simulink model "TST_PthSet_TrqCalc"  (R2016b)
settings: Solver=FixedStepDiscrete  StartTime=0.0  StopTime=simTime  FixedStep=sampleTime  RelTol=1e-3
values from neighbouring files (symbols this model uses):
  testCase = 1    [initTST_PthSet_TrqCalc_001.m]    (also in initTST_PthSet_TrqCalc_002.m = 2; initTST_PthSet_TrqCalc_003.m = 3)
libraries: simulink x17, UnitTest_Lib x12
settings Model: Creator=zhengjinyan  LastModifiedBy=zhengjinyan
settings DebuggingCC: SignalRangeChecking=error

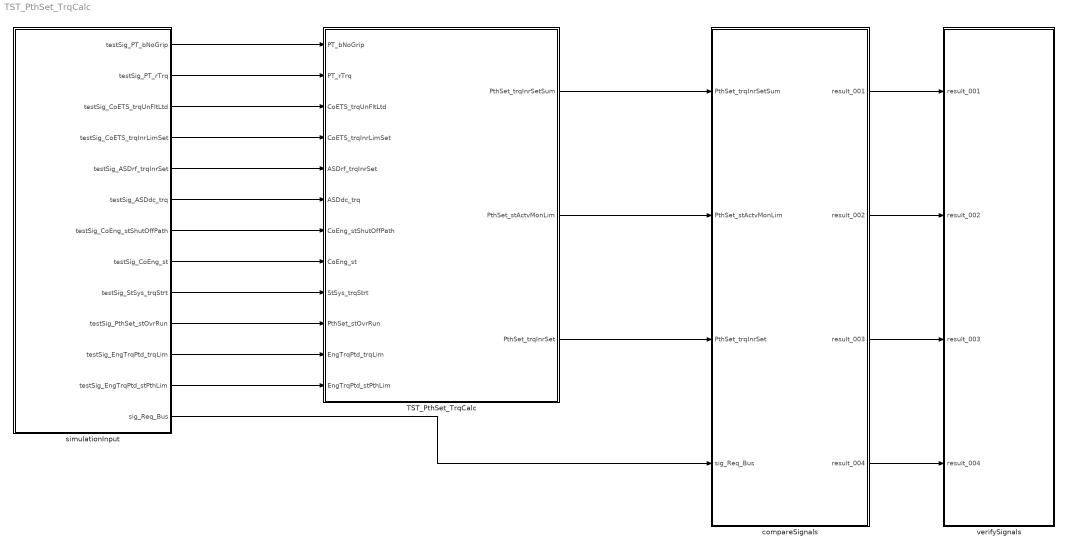
== system TST_PthSet_TrqCalc ==
  TST_PthSet_TrqCalc : Subsystem
  compareSignals : Subsystem
  simulationInput : Subsystem
  verifySignals : Subsystem
  wires:
  simulationInput/1(testSig_PT_bNoGrip) -> TST_PthSet_TrqCalc/1(PT_bNoGrip)
  simulationInput/2(testSig_PT_rTrq) -> TST_PthSet_TrqCalc/2(PT_rTrq)
  simulationInput/3(testSig_CoETS_trqUnFltLtd) -> TST_PthSet_TrqCalc/3(CoETS_trqUnFltLtd)
  simulationInput/4(testSig_CoETS_trqInrLimSet) -> TST_PthSet_TrqCalc/4(CoETS_trqInrLimSet)
  simulationInput/5(testSig_ASDrf_trqInrSet) -> TST_PthSet_TrqCalc/5(ASDrf_trqInrSet)
  simulationInput/6(testSig_ASDdc_trq) -> TST_PthSet_TrqCalc/6(ASDdc_trq)
  simulationInput/7(testSig_CoEng_stShutOffPath) -> TST_PthSet_TrqCalc/7(CoEng_stShutOffPath)
  simulationInput/8(testSig_CoEng_st) -> TST_PthSet_TrqCalc/8(CoEng_st)
  simulationInput/9(testSig_StSys_trqStrt) -> TST_PthSet_TrqCalc/9(StSys_trqStrt)
  simulationInput/10(testSig_PthSet_stOvrRun) -> TST_PthSet_TrqCalc/10(PthSet_stOvrRun)
  simulationInput/11(testSig_EngTrqPtd_trqLim) -> TST_PthSet_TrqCalc/11(EngTrqPtd_trqLim)
  simulationInput/12(testSig_EngTrqPtd_stPthLim) -> TST_PthSet_TrqCalc/12(EngTrqPtd_stPthLim)
  TST_PthSet_TrqCalc/1(PthSet_trqInrSetSum) -> compareSignals/1(PthSet_trqInrSetSum)
  TST_PthSet_TrqCalc/2(PthSet_stActvMonLim) -> compareSignals/2(PthSet_stActvMonLim)
  TST_PthSet_TrqCalc/3(PthSet_trqInrSet) -> compareSignals/3(PthSet_trqInrSet)
  simulationInput/13(sig_Req_Bus) -> compareSignals/4(sig_Req_Bus)
  compareSignals/1(result_001) -> verifySignals/1(result_001)
  compareSignals/2(result_002) -> verifySignals/2(result_002)
  compareSignals/3(result_003) -> verifySignals/3(result_003)
  compareSignals/4(result_004) -> verifySignals/4(result_004)

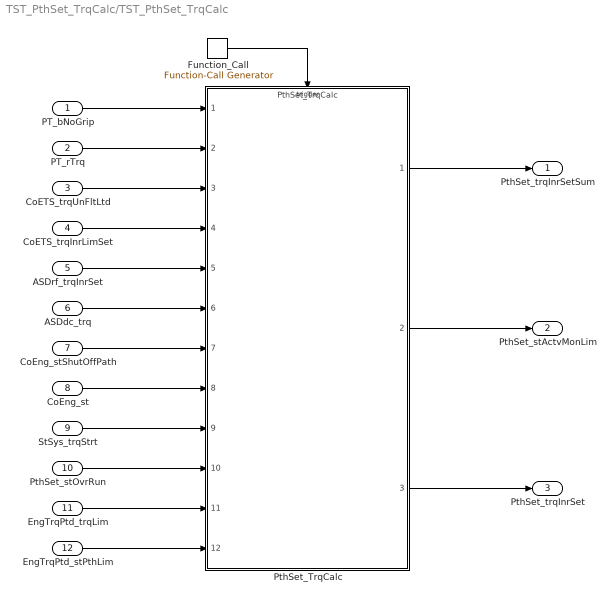
== system TST_PthSet_TrqCalc/TST_PthSet_TrqCalc ==
  PT_bNoGrip : Inport
  PT_rTrq : Inport  Port=2
  CoETS_trqUnFltLtd : Inport  Port=3
  CoETS_trqInrLimSet : Inport  Port=4
  ASDrf_trqInrSet : Inport  Port=5
  ASDdc_trq : Inport  Port=6
  CoEng_stShutOffPath : Inport  Port=7
  CoEng_st : Inport  Port=8
  StSys_trqStrt : Inport  Port=9
  PthSet_stOvrRun : Inport  Port=10
  EngTrqPtd_trqLim : Inport  Port=11
  EngTrqPtd_stPthLim : Inport  Port=12
  Function_Call : simulink/Ports & Subsystems/Function-Call Generator  sample_time=sampleTime  numberOfIterations=1
  PthSet_TrqCalc : ModelReference  ModelNameDialog=PthSet_TrqCalc  SimulationMode=Normal  ModelReferenceVersion=1.11  TriggerPortName=function  TriggerPortTriggerType=function-call  TriggerPortStatesWhenEnabling=held
  PthSet_trqInrSetSum : Outport
  PthSet_stActvMonLim : Outport  Port=2
  PthSet_trqInrSet : Outport  Port=3
  wires:
  Function_Call/1 -> PthSet_TrqCalc/Trigger
  PT_bNoGrip/1 -> PthSet_TrqCalc/1
  PT_rTrq/1 -> PthSet_TrqCalc/2
  CoETS_trqUnFltLtd/1 -> PthSet_TrqCalc/3
  CoETS_trqInrLimSet/1 -> PthSet_TrqCalc/4
  ASDrf_trqInrSet/1 -> PthSet_TrqCalc/5
  ASDdc_trq/1 -> PthSet_TrqCalc/6
  CoEng_stShutOffPath/1 -> PthSet_TrqCalc/7
  CoEng_st/1 -> PthSet_TrqCalc/8
  StSys_trqStrt/1 -> PthSet_TrqCalc/9
  PthSet_stOvrRun/1 -> PthSet_TrqCalc/10
  EngTrqPtd_trqLim/1 -> PthSet_TrqCalc/11
  EngTrqPtd_stPthLim/1 -> PthSet_TrqCalc/12
  PthSet_TrqCalc/1 -> PthSet_trqInrSetSum/1
  PthSet_TrqCalc/2 -> PthSet_stActvMonLim/1
  PthSet_TrqCalc/3 -> PthSet_trqInrSet/1

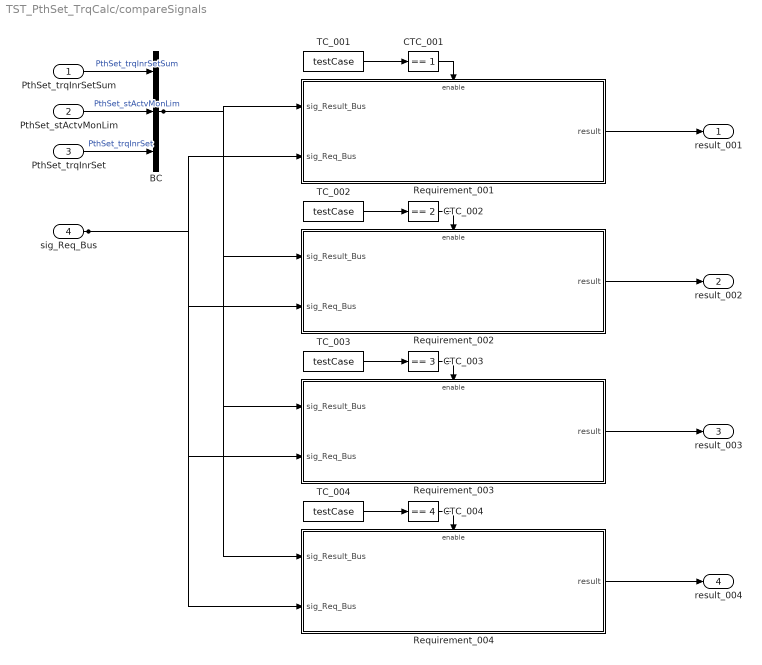
== system TST_PthSet_TrqCalc/compareSignals ==
  PthSet_trqInrSetSum : Inport
  PthSet_stActvMonLim : Inport  Port=2
  PthSet_trqInrSet : Inport  Port=3
  sig_Req_Bus : Inport  Port=4
  BC : BusCreator  Inputs=3
  CTC_001 : simulink/Logic and Bit Operations/Compare To Constant  relop===  const=1  OutDataTypeStr=boolean
  CTC_002 : simulink/Logic and Bit Operations/Compare To Constant  relop===  const=2  OutDataTypeStr=boolean
  CTC_003 : simulink/Logic and Bit Operations/Compare To Constant  relop===  const=3  OutDataTypeStr=boolean
  CTC_004 : simulink/Logic and Bit Operations/Compare To Constant  relop===  const=4  OutDataTypeStr=boolean
  Requirement_001 : Subsystem
  Requirement_002 : Subsystem
  Requirement_003 : Subsystem
  Requirement_004 : Subsystem
  TC_001 : Constant  Value=testCase
  TC_002 : Constant  Value=testCase
  TC_003 : Constant  Value=testCase
  TC_004 : Constant  Value=testCase
  result_001 : Outport
  result_002 : Outport  Port=2
  result_003 : Outport  Port=3
  result_004 : Outport  Port=4
  wires:
  PthSet_trqInrSetSum/1 -> BC/1  "PthSet_trqInrSetSum"
  PthSet_stActvMonLim/1 -> BC/2  "PthSet_stActvMonLim"
  PthSet_trqInrSet/1 -> BC/3  "PthSet_trqInrSet"
  TC_001/1 -> CTC_001/1
  CTC_001/1 -> Requirement_001/Enable
  sig_Req_Bus/1 -> Requirement_001/2(sig_Req_Bus), Requirement_002/2(sig_Req_Bus), Requirement_003/2(sig_Req_Bus), Requirement_004/2(sig_Req_Bus)
  BC/1 -> Requirement_001/1(sig_Result_Bus), Requirement_002/1(sig_Result_Bus), Requirement_003/1(sig_Result_Bus), Requirement_004/1(sig_Result_Bus)
  Requirement_001/1(result) -> result_001/1
  TC_002/1 -> CTC_002/1
  CTC_002/1 -> Requirement_002/Enable
  Requirement_002/1(result) -> result_002/1
  TC_003/1 -> CTC_003/1
  CTC_003/1 -> Requirement_003/Enable
  Requirement_003/1(result) -> result_003/1
  TC_004/1 -> CTC_004/1
  CTC_004/1 -> Requirement_004/Enable
  Requirement_004/1(result) -> result_004/1

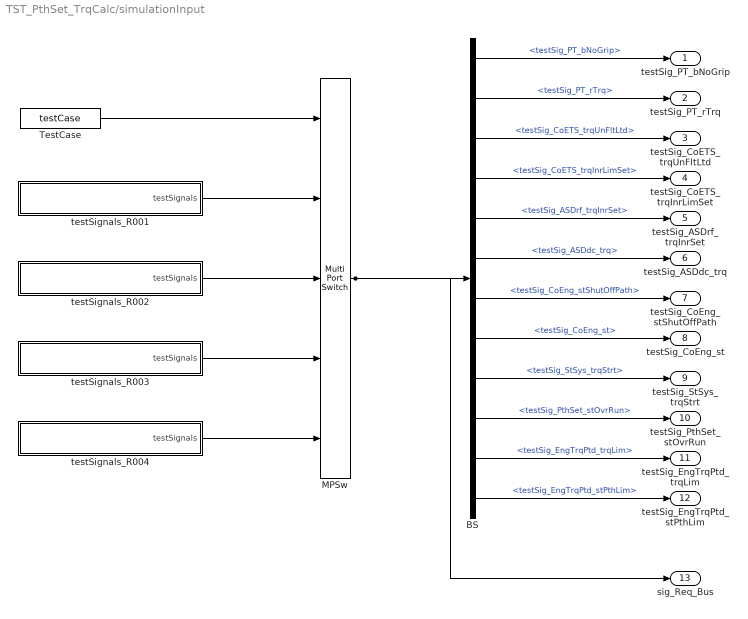
== system TST_PthSet_TrqCalc/simulationInput ==
  BS : BusSelector  OutputSignals=testSig_PT_bNoGrip,testSig_PT_rTrq,testSig_CoETS_trqUnFltLtd,testSig_CoETS_trqInrLimSet,testSig_ASDrf_trqInrSet,testSig_ASDdc_trq,testSig_CoEng_stShutOffPath,testSig_CoEng_st,testSig_StSys_trqStrt,testSig_PthSet_stOvrRun,testSig_EngTrqPtd_trqLim,testSig_EngTrqPtd_stPthLim
  MPSw : MultiPortSwitch  Inputs=4  SaturateOnIntegerOverflow=on  InputSameDT=on
  TestCase : Constant  Value=testCase
  testSignals_R001 : Subsystem
  testSignals_R002 : Subsystem
  testSignals_R003 : Subsystem
  testSignals_R004 : Subsystem
  testSig_PT_bNoGrip : Outport
  testSig_PT_rTrq : Outport  Port=2
  testSig_CoETS_trqUnFltLtd : Outport  Port=3
  testSig_CoETS_trqInrLimSet : Outport  Port=4
  testSig_ASDrf_trqInrSet : Outport  Port=5
  testSig_ASDdc_trq : Outport  Port=6
  testSig_CoEng_stShutOffPath : Outport  Port=7
  testSig_CoEng_st : Outport  Port=8
  testSig_StSys_trqStrt : Outport  Port=9
  testSig_PthSet_stOvrRun : Outport  Port=10
  testSig_EngTrqPtd_trqLim : Outport  Port=11
  testSig_EngTrqPtd_stPthLim : Outport  Port=12
  sig_Req_Bus : Outport  Port=13
  wires:
  BS/1 -> testSig_PT_bNoGrip/1  "<testSig_PT_bNoGrip>"
  BS/2 -> testSig_PT_rTrq/1  "<testSig_PT_rTrq>"
  BS/3 -> testSig_CoETS_trqUnFltLtd/1  "<testSig_CoETS_trqUnFltLtd>"
  BS/4 -> testSig_CoETS_trqInrLimSet/1  "<testSig_CoETS_trqInrLimSet>"
  BS/5 -> testSig_ASDrf_trqInrSet/1  "<testSig_ASDrf_trqInrSet>"
  BS/6 -> testSig_ASDdc_trq/1  "<testSig_ASDdc_trq>"
  BS/7 -> testSig_CoEng_stShutOffPath/1  "<testSig_CoEng_stShutOffPath>"
  BS/8 -> testSig_CoEng_st/1  "<testSig_CoEng_st>"
  BS/9 -> testSig_StSys_trqStrt/1  "<testSig_StSys_trqStrt>"
  BS/10 -> testSig_PthSet_stOvrRun/1  "<testSig_PthSet_stOvrRun>"
  BS/11 -> testSig_EngTrqPtd_trqLim/1  "<testSig_EngTrqPtd_trqLim>"
  BS/12 -> testSig_EngTrqPtd_stPthLim/1  "<testSig_EngTrqPtd_stPthLim>"
  MPSw/1 -> BS/1, sig_Req_Bus/1
  TestCase/1 -> MPSw/1
  testSignals_R001/1(testSignals) -> MPSw/2
  testSignals_R002/1(testSignals) -> MPSw/3
  testSignals_R003/1(testSignals) -> MPSw/4
  testSignals_R004/1(testSignals) -> MPSw/5

== system TST_PthSet_TrqCalc/verifySignals ==
  result_001 : Inport
  result_002 : Inport  Port=2
  result_003 : Inport  Port=3
  result_004 : Inport  Port=4
  Assertion_001 : Assertion  Enabled=off
  Assertion_002 : Assertion  Enabled=off
  Assertion_003 : Assertion  Enabled=off
  Assertion_004 : Assertion  Enabled=off
  wires:
  result_001/1 -> Assertion_001/1
  result_002/1 -> Assertion_002/1
  result_003/1 -> Assertion_003/1
  result_004/1 -> Assertion_004/1

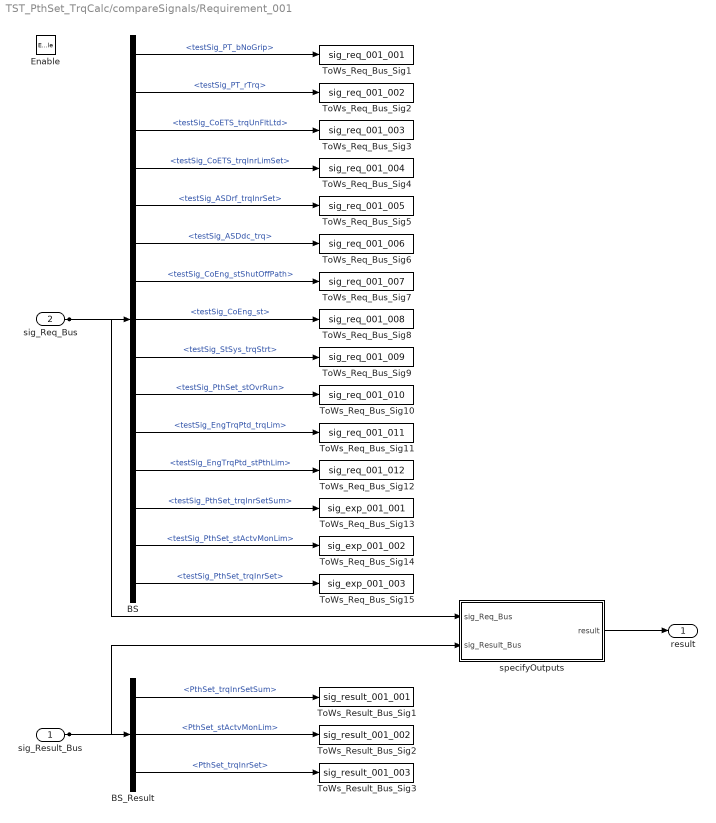
== system TST_PthSet_TrqCalc/compareSignals/Requirement_001 ==
  sig_Result_Bus : Inport
  sig_Req_Bus : Inport  Port=2
  Enable : EnablePort
  BS : BusSelector  OutputSignals=testSig_PT_bNoGrip,testSig_PT_rTrq,testSig_CoETS_trqUnFltLtd,testSig_CoETS_trqInrLimSet,testSig_ASDrf_trqInrSet,testSig_ASDdc_trq,testSig_CoEng_stShutOffPath,testSig_CoEng_st,testSig_StSys_trqStrt,testSig_PthSet_stOvrRun,testSig_EngTrqPtd_trqLim,testSig_EngTrqPtd_stPthLim,testSig_PthSet_trqInrSetSum,testSig_PthSet_stActvMonLim,testSig_PthSet_trqInrSet
  BS_Result : BusSelector  OutputSignals=PthSet_trqInrSetSum,PthSet_stActvMonLim,PthSet_trqInrSet
  ToWs_Req_Bus_Sig1 : ToWorkspace  VariableName=sig_req_001_001  SaveFormat=Structure With Time
  ToWs_Req_Bus_Sig10 : ToWorkspace  VariableName=sig_req_001_010  SaveFormat=Structure With Time
  ToWs_Req_Bus_Sig11 : ToWorkspace  VariableName=sig_req_001_011  SaveFormat=Structure With Time
  ToWs_Req_Bus_Sig12 : ToWorkspace  VariableName=sig_req_001_012  SaveFormat=Structure With Time
  ToWs_Req_Bus_Sig13 : ToWorkspace  VariableName=sig_exp_001_001  SaveFormat=Structure With Time
  ToWs_Req_Bus_Sig14 : ToWorkspace  VariableName=sig_exp_001_002  SaveFormat=Structure With Time
  ToWs_Req_Bus_Sig15 : ToWorkspace  VariableName=sig_exp_001_003  SaveFormat=Structure With Time
  ToWs_Req_Bus_Sig2 : ToWorkspace  VariableName=sig_req_001_002  SaveFormat=Structure With Time
  ToWs_Req_Bus_Sig3 : ToWorkspace  VariableName=sig_req_001_003  SaveFormat=Structure With Time
  ToWs_Req_Bus_Sig4 : ToWorkspace  VariableName=sig_req_001_004  SaveFormat=Structure With Time
  ToWs_Req_Bus_Sig5 : ToWorkspace  VariableName=sig_req_001_005  SaveFormat=Structure With Time
  ToWs_Req_Bus_Sig6 : ToWorkspace  VariableName=sig_req_001_006  SaveFormat=Structure With Time
  ToWs_Req_Bus_Sig7 : ToWorkspace  VariableName=sig_req_001_007  SaveFormat=Structure With Time
  ToWs_Req_Bus_Sig8 : ToWorkspace  VariableName=sig_req_001_008  SaveFormat=Structure With Time
  ToWs_Req_Bus_Sig9 : ToWorkspace  VariableName=sig_req_001_009  SaveFormat=Structure With Time
  ToWs_Result_Bus_Sig1 : ToWorkspace  VariableName=sig_result_001_001  SaveFormat=Structure With Time
  ToWs_Result_Bus_Sig2 : ToWorkspace  VariableName=sig_result_001_002  SaveFormat=Structure With Time
  ToWs_Result_Bus_Sig3 : ToWorkspace  VariableName=sig_result_001_003  SaveFormat=Structure With Time
  specifyOutputs : Subsystem
  result : Outport
  wires:
  sig_Req_Bus/1 -> BS/1, specifyOutputs/1(sig_Req_Bus)
  BS/1 -> ToWs_Req_Bus_Sig1/1  "<testSig_PT_bNoGrip>"
  BS/2 -> ToWs_Req_Bus_Sig2/1  "<testSig_PT_rTrq>"
  BS/3 -> ToWs_Req_Bus_Sig3/1  "<testSig_CoETS_trqUnFltLtd>"
  BS/4 -> ToWs_Req_Bus_Sig4/1  "<testSig_CoETS_trqInrLimSet>"
  BS/5 -> ToWs_Req_Bus_Sig5/1  "<testSig_ASDrf_trqInrSet>"
  BS/6 -> ToWs_Req_Bus_Sig6/1  "<testSig_ASDdc_trq>"
  BS/7 -> ToWs_Req_Bus_Sig7/1  "<testSig_CoEng_stShutOffPath>"
  BS/8 -> ToWs_Req_Bus_Sig8/1  "<testSig_CoEng_st>"
  BS/9 -> ToWs_Req_Bus_Sig9/1  "<testSig_StSys_trqStrt>"
  BS/10 -> ToWs_Req_Bus_Sig10/1  "<testSig_PthSet_stOvrRun>"
  BS/11 -> ToWs_Req_Bus_Sig11/1  "<testSig_EngTrqPtd_trqLim>"
  BS/12 -> ToWs_Req_Bus_Sig12/1  "<testSig_EngTrqPtd_stPthLim>"
  BS/13 -> ToWs_Req_Bus_Sig13/1  "<testSig_PthSet_trqInrSetSum>"
  BS/14 -> ToWs_Req_Bus_Sig14/1  "<testSig_PthSet_stActvMonLim>"
  BS/15 -> ToWs_Req_Bus_Sig15/1  "<testSig_PthSet_trqInrSet>"
  sig_Result_Bus/1 -> BS_Result/1, specifyOutputs/2(sig_Result_Bus)
  BS_Result/1 -> ToWs_Result_Bus_Sig1/1  "<PthSet_trqInrSetSum>"
  BS_Result/2 -> ToWs_Result_Bus_Sig2/1  "<PthSet_stActvMonLim>"
  BS_Result/3 -> ToWs_Result_Bus_Sig3/1  "<PthSet_trqInrSet>"
  specifyOutputs/1(result) -> result/1

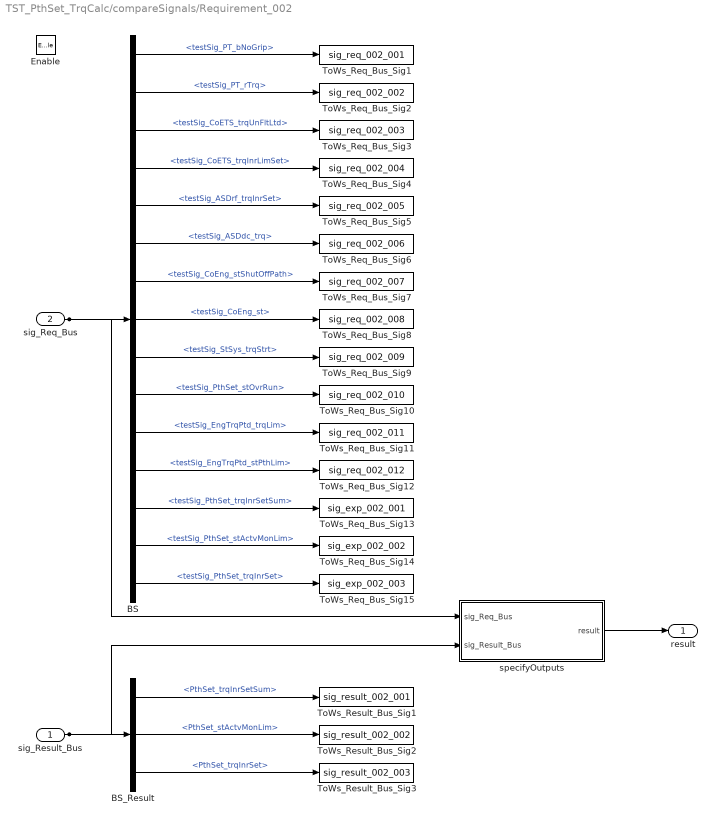
== system TST_PthSet_TrqCalc/compareSignals/Requirement_002 ==
  sig_Result_Bus : Inport
  sig_Req_Bus : Inport  Port=2
  Enable : EnablePort
  BS : BusSelector  OutputSignals=testSig_PT_bNoGrip,testSig_PT_rTrq,testSig_CoETS_trqUnFltLtd,testSig_CoETS_trqInrLimSet,testSig_ASDrf_trqInrSet,testSig_ASDdc_trq,testSig_CoEng_stShutOffPath,testSig_CoEng_st,testSig_StSys_trqStrt,testSig_PthSet_stOvrRun,testSig_EngTrqPtd_trqLim,testSig_EngTrqPtd_stPthLim,testSig_PthSet_trqInrSetSum,testSig_PthSet_stActvMonLim,testSig_PthSet_trqInrSet
  BS_Result : BusSelector  OutputSignals=PthSet_trqInrSetSum,PthSet_stActvMonLim,PthSet_trqInrSet
  ToWs_Req_Bus_Sig1 : ToWorkspace  VariableName=sig_req_002_001  SaveFormat=Structure With Time
  ToWs_Req_Bus_Sig10 : ToWorkspace  VariableName=sig_req_002_010  SaveFormat=Structure With Time
  ToWs_Req_Bus_Sig11 : ToWorkspace  VariableName=sig_req_002_011  SaveFormat=Structure With Time
  ToWs_Req_Bus_Sig12 : ToWorkspace  VariableName=sig_req_002_012  SaveFormat=Structure With Time
  ToWs_Req_Bus_Sig13 : ToWorkspace  VariableName=sig_exp_002_001  SaveFormat=Structure With Time
  ToWs_Req_Bus_Sig14 : ToWorkspace  VariableName=sig_exp_002_002  SaveFormat=Structure With Time
  ToWs_Req_Bus_Sig15 : ToWorkspace  VariableName=sig_exp_002_003  SaveFormat=Structure With Time
  ToWs_Req_Bus_Sig2 : ToWorkspace  VariableName=sig_req_002_002  SaveFormat=Structure With Time
  ToWs_Req_Bus_Sig3 : ToWorkspace  VariableName=sig_req_002_003  SaveFormat=Structure With Time
  ToWs_Req_Bus_Sig4 : ToWorkspace  VariableName=sig_req_002_004  SaveFormat=Structure With Time
  ToWs_Req_Bus_Sig5 : ToWorkspace  VariableName=sig_req_002_005  SaveFormat=Structure With Time
  ToWs_Req_Bus_Sig6 : ToWorkspace  VariableName=sig_req_002_006  SaveFormat=Structure With Time
  ToWs_Req_Bus_Sig7 : ToWorkspace  VariableName=sig_req_002_007  SaveFormat=Structure With Time
  ToWs_Req_Bus_Sig8 : ToWorkspace  VariableName=sig_req_002_008  SaveFormat=Structure With Time
  ToWs_Req_Bus_Sig9 : ToWorkspace  VariableName=sig_req_002_009  SaveFormat=Structure With Time
  ToWs_Result_Bus_Sig1 : ToWorkspace  VariableName=sig_result_002_001  SaveFormat=Structure With Time
  ToWs_Result_Bus_Sig2 : ToWorkspace  VariableName=sig_result_002_002  SaveFormat=Structure With Time
  ToWs_Result_Bus_Sig3 : ToWorkspace  VariableName=sig_result_002_003  SaveFormat=Structure With Time
  specifyOutputs : Subsystem
  result : Outport
  wires:
  sig_Req_Bus/1 -> BS/1, specifyOutputs/1(sig_Req_Bus)
  BS/1 -> ToWs_Req_Bus_Sig1/1  "<testSig_PT_bNoGrip>"
  BS/2 -> ToWs_Req_Bus_Sig2/1  "<testSig_PT_rTrq>"
  BS/3 -> ToWs_Req_Bus_Sig3/1  "<testSig_CoETS_trqUnFltLtd>"
  BS/4 -> ToWs_Req_Bus_Sig4/1  "<testSig_CoETS_trqInrLimSet>"
  BS/5 -> ToWs_Req_Bus_Sig5/1  "<testSig_ASDrf_trqInrSet>"
  BS/6 -> ToWs_Req_Bus_Sig6/1  "<testSig_ASDdc_trq>"
  BS/7 -> ToWs_Req_Bus_Sig7/1  "<testSig_CoEng_stShutOffPath>"
  BS/8 -> ToWs_Req_Bus_Sig8/1  "<testSig_CoEng_st>"
  BS/9 -> ToWs_Req_Bus_Sig9/1  "<testSig_StSys_trqStrt>"
  BS/10 -> ToWs_Req_Bus_Sig10/1  "<testSig_PthSet_stOvrRun>"
  BS/11 -> ToWs_Req_Bus_Sig11/1  "<testSig_EngTrqPtd_trqLim>"
  BS/12 -> ToWs_Req_Bus_Sig12/1  "<testSig_EngTrqPtd_stPthLim>"
  BS/13 -> ToWs_Req_Bus_Sig13/1  "<testSig_PthSet_trqInrSetSum>"
  BS/14 -> ToWs_Req_Bus_Sig14/1  "<testSig_PthSet_stActvMonLim>"
  BS/15 -> ToWs_Req_Bus_Sig15/1  "<testSig_PthSet_trqInrSet>"
  sig_Result_Bus/1 -> BS_Result/1, specifyOutputs/2(sig_Result_Bus)
  BS_Result/1 -> ToWs_Result_Bus_Sig1/1  "<PthSet_trqInrSetSum>"
  BS_Result/2 -> ToWs_Result_Bus_Sig2/1  "<PthSet_stActvMonLim>"
  BS_Result/3 -> ToWs_Result_Bus_Sig3/1  "<PthSet_trqInrSet>"
  specifyOutputs/1(result) -> result/1

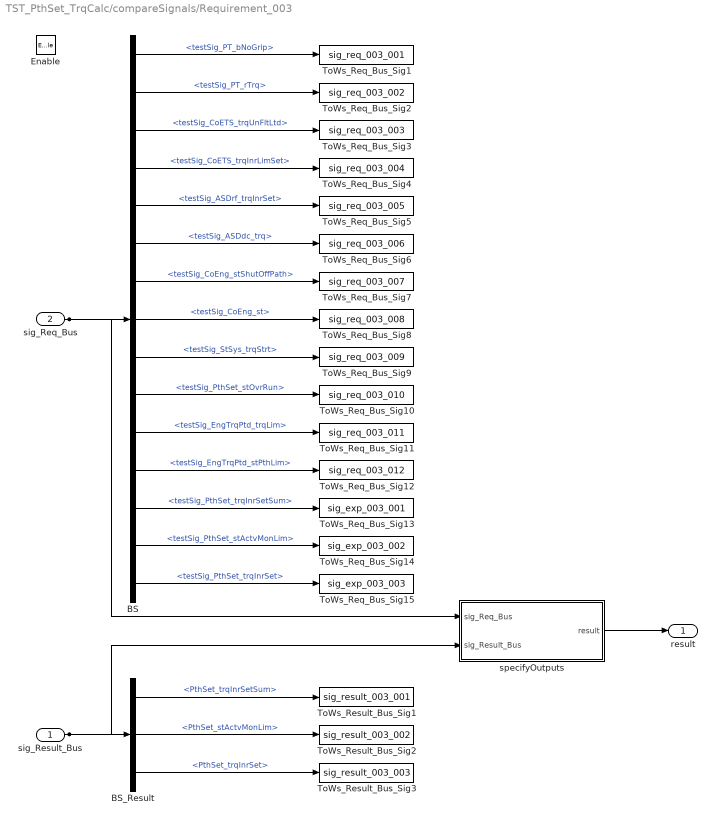
== system TST_PthSet_TrqCalc/compareSignals/Requirement_003 ==
  sig_Result_Bus : Inport
  sig_Req_Bus : Inport  Port=2
  Enable : EnablePort
  BS : BusSelector  OutputSignals=testSig_PT_bNoGrip,testSig_PT_rTrq,testSig_CoETS_trqUnFltLtd,testSig_CoETS_trqInrLimSet,testSig_ASDrf_trqInrSet,testSig_ASDdc_trq,testSig_CoEng_stShutOffPath,testSig_CoEng_st,testSig_StSys_trqStrt,testSig_PthSet_stOvrRun,testSig_EngTrqPtd_trqLim,testSig_EngTrqPtd_stPthLim,testSig_PthSet_trqInrSetSum,testSig_PthSet_stActvMonLim,testSig_PthSet_trqInrSet
  BS_Result : BusSelector  OutputSignals=PthSet_trqInrSetSum,PthSet_stActvMonLim,PthSet_trqInrSet
  ToWs_Req_Bus_Sig1 : ToWorkspace  VariableName=sig_req_003_001  SaveFormat=Structure With Time
  ToWs_Req_Bus_Sig10 : ToWorkspace  VariableName=sig_req_003_010  SaveFormat=Structure With Time
  ToWs_Req_Bus_Sig11 : ToWorkspace  VariableName=sig_req_003_011  SaveFormat=Structure With Time
  ToWs_Req_Bus_Sig12 : ToWorkspace  VariableName=sig_req_003_012  SaveFormat=Structure With Time
  ToWs_Req_Bus_Sig13 : ToWorkspace  VariableName=sig_exp_003_001  SaveFormat=Structure With Time
  ToWs_Req_Bus_Sig14 : ToWorkspace  VariableName=sig_exp_003_002  SaveFormat=Structure With Time
  ToWs_Req_Bus_Sig15 : ToWorkspace  VariableName=sig_exp_003_003  SaveFormat=Structure With Time
  ToWs_Req_Bus_Sig2 : ToWorkspace  VariableName=sig_req_003_002  SaveFormat=Structure With Time
  ToWs_Req_Bus_Sig3 : ToWorkspace  VariableName=sig_req_003_003  SaveFormat=Structure With Time
  ToWs_Req_Bus_Sig4 : ToWorkspace  VariableName=sig_req_003_004  SaveFormat=Structure With Time
  ToWs_Req_Bus_Sig5 : ToWorkspace  VariableName=sig_req_003_005  SaveFormat=Structure With Time
  ToWs_Req_Bus_Sig6 : ToWorkspace  VariableName=sig_req_003_006  SaveFormat=Structure With Time
  ToWs_Req_Bus_Sig7 : ToWorkspace  VariableName=sig_req_003_007  SaveFormat=Structure With Time
  ToWs_Req_Bus_Sig8 : ToWorkspace  VariableName=sig_req_003_008  SaveFormat=Structure With Time
  ToWs_Req_Bus_Sig9 : ToWorkspace  VariableName=sig_req_003_009  SaveFormat=Structure With Time
  ToWs_Result_Bus_Sig1 : ToWorkspace  VariableName=sig_result_003_001  SaveFormat=Structure With Time
  ToWs_Result_Bus_Sig2 : ToWorkspace  VariableName=sig_result_003_002  SaveFormat=Structure With Time
  ToWs_Result_Bus_Sig3 : ToWorkspace  VariableName=sig_result_003_003  SaveFormat=Structure With Time
  specifyOutputs : Subsystem
  result : Outport
  wires:
  sig_Req_Bus/1 -> BS/1, specifyOutputs/1(sig_Req_Bus)
  BS/1 -> ToWs_Req_Bus_Sig1/1  "<testSig_PT_bNoGrip>"
  BS/2 -> ToWs_Req_Bus_Sig2/1  "<testSig_PT_rTrq>"
  BS/3 -> ToWs_Req_Bus_Sig3/1  "<testSig_CoETS_trqUnFltLtd>"
  BS/4 -> ToWs_Req_Bus_Sig4/1  "<testSig_CoETS_trqInrLimSet>"
  BS/5 -> ToWs_Req_Bus_Sig5/1  "<testSig_ASDrf_trqInrSet>"
  BS/6 -> ToWs_Req_Bus_Sig6/1  "<testSig_ASDdc_trq>"
  BS/7 -> ToWs_Req_Bus_Sig7/1  "<testSig_CoEng_stShutOffPath>"
  BS/8 -> ToWs_Req_Bus_Sig8/1  "<testSig_CoEng_st>"
  BS/9 -> ToWs_Req_Bus_Sig9/1  "<testSig_StSys_trqStrt>"
  BS/10 -> ToWs_Req_Bus_Sig10/1  "<testSig_PthSet_stOvrRun>"
  BS/11 -> ToWs_Req_Bus_Sig11/1  "<testSig_EngTrqPtd_trqLim>"
  BS/12 -> ToWs_Req_Bus_Sig12/1  "<testSig_EngTrqPtd_stPthLim>"
  BS/13 -> ToWs_Req_Bus_Sig13/1  "<testSig_PthSet_trqInrSetSum>"
  BS/14 -> ToWs_Req_Bus_Sig14/1  "<testSig_PthSet_stActvMonLim>"
  BS/15 -> ToWs_Req_Bus_Sig15/1  "<testSig_PthSet_trqInrSet>"
  sig_Result_Bus/1 -> BS_Result/1, specifyOutputs/2(sig_Result_Bus)
  BS_Result/1 -> ToWs_Result_Bus_Sig1/1  "<PthSet_trqInrSetSum>"
  BS_Result/2 -> ToWs_Result_Bus_Sig2/1  "<PthSet_stActvMonLim>"
  BS_Result/3 -> ToWs_Result_Bus_Sig3/1  "<PthSet_trqInrSet>"
  specifyOutputs/1(result) -> result/1

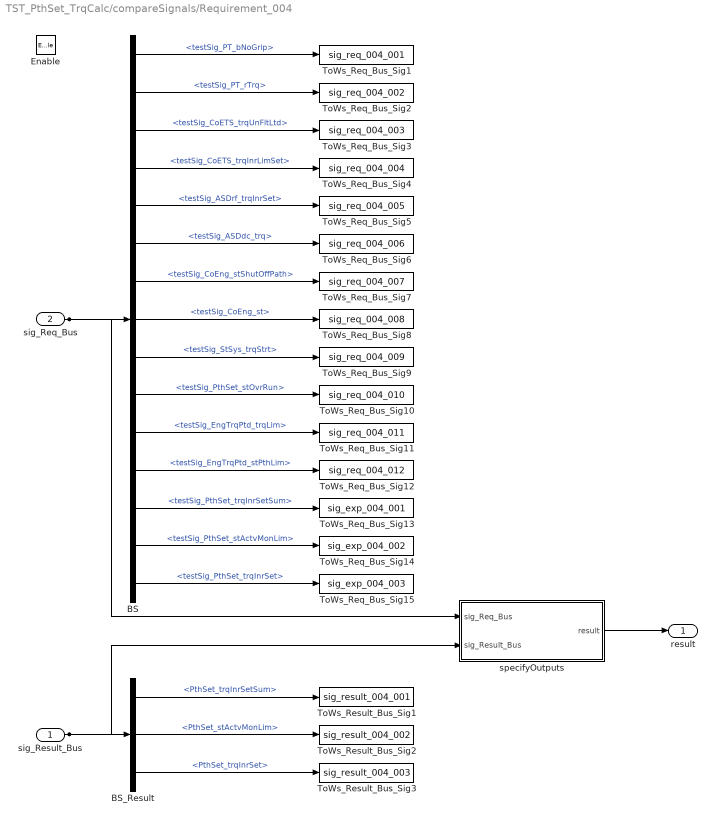
== system TST_PthSet_TrqCalc/compareSignals/Requirement_004 ==
  sig_Result_Bus : Inport
  sig_Req_Bus : Inport  Port=2
  Enable : EnablePort
  BS : BusSelector  OutputSignals=testSig_PT_bNoGrip,testSig_PT_rTrq,testSig_CoETS_trqUnFltLtd,testSig_CoETS_trqInrLimSet,testSig_ASDrf_trqInrSet,testSig_ASDdc_trq,testSig_CoEng_stShutOffPath,testSig_CoEng_st,testSig_StSys_trqStrt,testSig_PthSet_stOvrRun,testSig_EngTrqPtd_trqLim,testSig_EngTrqPtd_stPthLim,testSig_PthSet_trqInrSetSum,testSig_PthSet_stActvMonLim,testSig_PthSet_trqInrSet
  BS_Result : BusSelector  OutputSignals=PthSet_trqInrSetSum,PthSet_stActvMonLim,PthSet_trqInrSet
  ToWs_Req_Bus_Sig1 : ToWorkspace  VariableName=sig_req_004_001  SaveFormat=Structure With Time
  ToWs_Req_Bus_Sig10 : ToWorkspace  VariableName=sig_req_004_010  SaveFormat=Structure With Time
  ToWs_Req_Bus_Sig11 : ToWorkspace  VariableName=sig_req_004_011  SaveFormat=Structure With Time
  ToWs_Req_Bus_Sig12 : ToWorkspace  VariableName=sig_req_004_012  SaveFormat=Structure With Time
  ToWs_Req_Bus_Sig13 : ToWorkspace  VariableName=sig_exp_004_001  SaveFormat=Structure With Time
  ToWs_Req_Bus_Sig14 : ToWorkspace  VariableName=sig_exp_004_002  SaveFormat=Structure With Time
  ToWs_Req_Bus_Sig15 : ToWorkspace  VariableName=sig_exp_004_003  SaveFormat=Structure With Time
  ToWs_Req_Bus_Sig2 : ToWorkspace  VariableName=sig_req_004_002  SaveFormat=Structure With Time
  ToWs_Req_Bus_Sig3 : ToWorkspace  VariableName=sig_req_004_003  SaveFormat=Structure With Time
  ToWs_Req_Bus_Sig4 : ToWorkspace  VariableName=sig_req_004_004  SaveFormat=Structure With Time
  ToWs_Req_Bus_Sig5 : ToWorkspace  VariableName=sig_req_004_005  SaveFormat=Structure With Time
  ToWs_Req_Bus_Sig6 : ToWorkspace  VariableName=sig_req_004_006  SaveFormat=Structure With Time
  ToWs_Req_Bus_Sig7 : ToWorkspace  VariableName=sig_req_004_007  SaveFormat=Structure With Time
  ToWs_Req_Bus_Sig8 : ToWorkspace  VariableName=sig_req_004_008  SaveFormat=Structure With Time
  ToWs_Req_Bus_Sig9 : ToWorkspace  VariableName=sig_req_004_009  SaveFormat=Structure With Time
  ToWs_Result_Bus_Sig1 : ToWorkspace  VariableName=sig_result_004_001  SaveFormat=Structure With Time
  ToWs_Result_Bus_Sig2 : ToWorkspace  VariableName=sig_result_004_002  SaveFormat=Structure With Time
  ToWs_Result_Bus_Sig3 : ToWorkspace  VariableName=sig_result_004_003  SaveFormat=Structure With Time
  specifyOutputs : Subsystem
  result : Outport
  wires:
  sig_Req_Bus/1 -> BS/1, specifyOutputs/1(sig_Req_Bus)
  BS/1 -> ToWs_Req_Bus_Sig1/1  "<testSig_PT_bNoGrip>"
  BS/2 -> ToWs_Req_Bus_Sig2/1  "<testSig_PT_rTrq>"
  BS/3 -> ToWs_Req_Bus_Sig3/1  "<testSig_CoETS_trqUnFltLtd>"
  BS/4 -> ToWs_Req_Bus_Sig4/1  "<testSig_CoETS_trqInrLimSet>"
  BS/5 -> ToWs_Req_Bus_Sig5/1  "<testSig_ASDrf_trqInrSet>"
  BS/6 -> ToWs_Req_Bus_Sig6/1  "<testSig_ASDdc_trq>"
  BS/7 -> ToWs_Req_Bus_Sig7/1  "<testSig_CoEng_stShutOffPath>"
  BS/8 -> ToWs_Req_Bus_Sig8/1  "<testSig_CoEng_st>"
  BS/9 -> ToWs_Req_Bus_Sig9/1  "<testSig_StSys_trqStrt>"
  BS/10 -> ToWs_Req_Bus_Sig10/1  "<testSig_PthSet_stOvrRun>"
  BS/11 -> ToWs_Req_Bus_Sig11/1  "<testSig_EngTrqPtd_trqLim>"
  BS/12 -> ToWs_Req_Bus_Sig12/1  "<testSig_EngTrqPtd_stPthLim>"
  BS/13 -> ToWs_Req_Bus_Sig13/1  "<testSig_PthSet_trqInrSetSum>"
  BS/14 -> ToWs_Req_Bus_Sig14/1  "<testSig_PthSet_stActvMonLim>"
  BS/15 -> ToWs_Req_Bus_Sig15/1  "<testSig_PthSet_trqInrSet>"
  sig_Result_Bus/1 -> BS_Result/1, specifyOutputs/2(sig_Result_Bus)
  BS_Result/1 -> ToWs_Result_Bus_Sig1/1  "<PthSet_trqInrSetSum>"
  BS_Result/2 -> ToWs_Result_Bus_Sig2/1  "<PthSet_stActvMonLim>"
  BS_Result/3 -> ToWs_Result_Bus_Sig3/1  "<PthSet_trqInrSet>"
  specifyOutputs/1(result) -> result/1

== system TST_PthSet_TrqCalc/simulationInput/testSignals_R001 ==
  BC : BusCreator  Inputs=15
  spec_ASDdc_trq : FromWorkspace  VariableName=testSig_ASDdc_trq  Interpolate=off  OutputAfterFinalValue=Holding final value
  spec_ASDrf_trqInrSet : FromWorkspace  VariableName=testSig_ASDrf_trqInrSet  Interpolate=off  OutputAfterFinalValue=Holding final value
  spec_CoETS_trqInrLimSet : FromWorkspace  VariableName=testSig_CoETS_trqInrLimSet  Interpolate=off  OutputAfterFinalValue=Holding final value
  spec_CoETS_trqUnFltLtd : FromWorkspace  VariableName=testSig_CoETS_trqUnFltLtd  Interpolate=off  OutputAfterFinalValue=Holding final value
  spec_CoEng_st : FromWorkspace  VariableName=testSig_CoEng_st  Interpolate=off  OutputAfterFinalValue=Holding final value
  spec_CoEng_stShutOffPath : FromWorkspace  VariableName=testSig_CoEng_stShutOffPath  Interpolate=off  OutputAfterFinalValue=Holding final value
  spec_EngTrqPtd_stPthLim : FromWorkspace  VariableName=testSig_EngTrqPtd_stPthLim  Interpolate=off  OutputAfterFinalValue=Holding final value
  spec_EngTrqPtd_trqLim : FromWorkspace  VariableName=testSig_EngTrqPtd_trqLim  Interpolate=off  OutputAfterFinalValue=Holding final value
  spec_PT_bNoGrip : FromWorkspace  VariableName=testSig_PT_bNoGrip  Interpolate=off  OutputAfterFinalValue=Holding final value
  spec_PT_rTrq : FromWorkspace  VariableName=testSig_PT_rTrq  Interpolate=off  OutputAfterFinalValue=Holding final value
  spec_PthSet_stActvMonLim : FromWorkspace  VariableName=testSig_PthSet_stActvMonLim  Interpolate=off  OutputAfterFinalValue=Holding final value
  spec_PthSet_stOvrRun : FromWorkspace  VariableName=testSig_PthSet_stOvrRun  Interpolate=off  OutputAfterFinalValue=Holding final value
  spec_PthSet_trqInrSet : FromWorkspace  VariableName=testSig_PthSet_trqInrSet  Interpolate=off  OutputAfterFinalValue=Holding final value
  spec_PthSet_trqInrSetSum : FromWorkspace  VariableName=testSig_PthSet_trqInrSetSum  Interpolate=off  OutputAfterFinalValue=Holding final value
  spec_StSys_trqStrt : FromWorkspace  VariableName=testSig_StSys_trqStrt  Interpolate=off  OutputAfterFinalValue=Holding final value
  testSignals : Outport
  wires:
  BC/1 -> testSignals/1
  spec_PT_bNoGrip/1 -> BC/1  "testSig_PT_bNoGrip"
  spec_PT_rTrq/1 -> BC/2  "testSig_PT_rTrq"
  spec_CoETS_trqUnFltLtd/1 -> BC/3  "testSig_CoETS_trqUnFltLtd"
  spec_CoETS_trqInrLimSet/1 -> BC/4  "testSig_CoETS_trqInrLimSet"
  spec_ASDrf_trqInrSet/1 -> BC/5  "testSig_ASDrf_trqInrSet"
  spec_ASDdc_trq/1 -> BC/6  "testSig_ASDdc_trq"
  spec_CoEng_stShutOffPath/1 -> BC/7  "testSig_CoEng_stShutOffPath"
  spec_CoEng_st/1 -> BC/8  "testSig_CoEng_st"
  spec_StSys_trqStrt/1 -> BC/9  "testSig_StSys_trqStrt"
  spec_PthSet_stOvrRun/1 -> BC/10  "testSig_PthSet_stOvrRun"
  spec_EngTrqPtd_trqLim/1 -> BC/11  "testSig_EngTrqPtd_trqLim"
  spec_EngTrqPtd_stPthLim/1 -> BC/12  "testSig_EngTrqPtd_stPthLim"
  spec_PthSet_trqInrSetSum/1 -> BC/13  "testSig_PthSet_trqInrSetSum"
  spec_PthSet_stActvMonLim/1 -> BC/14  "testSig_PthSet_stActvMonLim"
  spec_PthSet_trqInrSet/1 -> BC/15  "testSig_PthSet_trqInrSet"

== system TST_PthSet_TrqCalc/simulationInput/testSignals_R002 ==
  BC : BusCreator  Inputs=15
  spec_ASDdc_trq : FromWorkspace  VariableName=testSig_ASDdc_trq  Interpolate=off  OutputAfterFinalValue=Holding final value
  spec_ASDrf_trqInrSet : FromWorkspace  VariableName=testSig_ASDrf_trqInrSet  Interpolate=off  OutputAfterFinalValue=Holding final value
  spec_CoETS_trqInrLimSet : FromWorkspace  VariableName=testSig_CoETS_trqInrLimSet  Interpolate=off  OutputAfterFinalValue=Holding final value
  spec_CoETS_trqUnFltLtd : FromWorkspace  VariableName=testSig_CoETS_trqUnFltLtd  Interpolate=off  OutputAfterFinalValue=Holding final value
  spec_CoEng_st : FromWorkspace  VariableName=testSig_CoEng_st  Interpolate=off  OutputAfterFinalValue=Holding final value
  spec_CoEng_stShutOffPath : FromWorkspace  VariableName=testSig_CoEng_stShutOffPath  Interpolate=off  OutputAfterFinalValue=Holding final value
  spec_EngTrqPtd_stPthLim : FromWorkspace  VariableName=testSig_EngTrqPtd_stPthLim  Interpolate=off  OutputAfterFinalValue=Holding final value
  spec_EngTrqPtd_trqLim : FromWorkspace  VariableName=testSig_EngTrqPtd_trqLim  Interpolate=off  OutputAfterFinalValue=Holding final value
  spec_PT_bNoGrip : FromWorkspace  VariableName=testSig_PT_bNoGrip  Interpolate=off  OutputAfterFinalValue=Holding final value
  spec_PT_rTrq : FromWorkspace  VariableName=testSig_PT_rTrq  Interpolate=off  OutputAfterFinalValue=Holding final value
  spec_PthSet_stActvMonLim : FromWorkspace  VariableName=testSig_PthSet_stActvMonLim  Interpolate=off  OutputAfterFinalValue=Holding final value
  spec_PthSet_stOvrRun : FromWorkspace  VariableName=testSig_PthSet_stOvrRun  Interpolate=off  OutputAfterFinalValue=Holding final value
  spec_PthSet_trqInrSet : FromWorkspace  VariableName=testSig_PthSet_trqInrSet  Interpolate=off  OutputAfterFinalValue=Holding final value
  spec_PthSet_trqInrSetSum : FromWorkspace  VariableName=testSig_PthSet_trqInrSetSum  Interpolate=off  OutputAfterFinalValue=Holding final value
  spec_StSys_trqStrt : FromWorkspace  VariableName=testSig_StSys_trqStrt  Interpolate=off  OutputAfterFinalValue=Holding final value
  testSignals : Outport
  wires:
  BC/1 -> testSignals/1
  spec_PT_bNoGrip/1 -> BC/1  "testSig_PT_bNoGrip"
  spec_PT_rTrq/1 -> BC/2  "testSig_PT_rTrq"
  spec_CoETS_trqUnFltLtd/1 -> BC/3  "testSig_CoETS_trqUnFltLtd"
  spec_CoETS_trqInrLimSet/1 -> BC/4  "testSig_CoETS_trqInrLimSet"
  spec_ASDrf_trqInrSet/1 -> BC/5  "testSig_ASDrf_trqInrSet"
  spec_ASDdc_trq/1 -> BC/6  "testSig_ASDdc_trq"
  spec_CoEng_stShutOffPath/1 -> BC/7  "testSig_CoEng_stShutOffPath"
  spec_CoEng_st/1 -> BC/8  "testSig_CoEng_st"
  spec_StSys_trqStrt/1 -> BC/9  "testSig_StSys_trqStrt"
  spec_PthSet_stOvrRun/1 -> BC/10  "testSig_PthSet_stOvrRun"
  spec_EngTrqPtd_trqLim/1 -> BC/11  "testSig_EngTrqPtd_trqLim"
  spec_EngTrqPtd_stPthLim/1 -> BC/12  "testSig_EngTrqPtd_stPthLim"
  spec_PthSet_trqInrSetSum/1 -> BC/13  "testSig_PthSet_trqInrSetSum"
  spec_PthSet_stActvMonLim/1 -> BC/14  "testSig_PthSet_stActvMonLim"
  spec_PthSet_trqInrSet/1 -> BC/15  "testSig_PthSet_trqInrSet"

== system TST_PthSet_TrqCalc/simulationInput/testSignals_R003 ==
  BC : BusCreator  Inputs=15
  spec_ASDdc_trq : FromWorkspace  VariableName=testSig_ASDdc_trq  Interpolate=off  OutputAfterFinalValue=Holding final value
  spec_ASDrf_trqInrSet : FromWorkspace  VariableName=testSig_ASDrf_trqInrSet  Interpolate=off  OutputAfterFinalValue=Holding final value
  spec_CoETS_trqInrLimSet : FromWorkspace  VariableName=testSig_CoETS_trqInrLimSet  Interpolate=off  OutputAfterFinalValue=Holding final value
  spec_CoETS_trqUnFltLtd : FromWorkspace  VariableName=testSig_CoETS_trqUnFltLtd  Interpolate=off  OutputAfterFinalValue=Holding final value
  spec_CoEng_st : FromWorkspace  VariableName=testSig_CoEng_st  Interpolate=off  OutputAfterFinalValue=Holding final value
  spec_CoEng_stShutOffPath : FromWorkspace  VariableName=testSig_CoEng_stShutOffPath  Interpolate=off  OutputAfterFinalValue=Holding final value
  spec_EngTrqPtd_stPthLim : FromWorkspace  VariableName=testSig_EngTrqPtd_stPthLim  Interpolate=off  OutputAfterFinalValue=Holding final value
  spec_EngTrqPtd_trqLim : FromWorkspace  VariableName=testSig_EngTrqPtd_trqLim  Interpolate=off  OutputAfterFinalValue=Holding final value
  spec_PT_bNoGrip : FromWorkspace  VariableName=testSig_PT_bNoGrip  Interpolate=off  OutputAfterFinalValue=Holding final value
  spec_PT_rTrq : FromWorkspace  VariableName=testSig_PT_rTrq  Interpolate=off  OutputAfterFinalValue=Holding final value
  spec_PthSet_stActvMonLim : FromWorkspace  VariableName=testSig_PthSet_stActvMonLim  Interpolate=off  OutputAfterFinalValue=Holding final value
  spec_PthSet_stOvrRun : FromWorkspace  VariableName=testSig_PthSet_stOvrRun  Interpolate=off  OutputAfterFinalValue=Holding final value
  spec_PthSet_trqInrSet : FromWorkspace  VariableName=testSig_PthSet_trqInrSet  Interpolate=off  OutputAfterFinalValue=Holding final value
  spec_PthSet_trqInrSetSum : FromWorkspace  VariableName=testSig_PthSet_trqInrSetSum  Interpolate=off  OutputAfterFinalValue=Holding final value
  spec_StSys_trqStrt : FromWorkspace  VariableName=testSig_StSys_trqStrt  Interpolate=off  OutputAfterFinalValue=Holding final value
  testSignals : Outport
  wires:
  BC/1 -> testSignals/1
  spec_PT_bNoGrip/1 -> BC/1  "testSig_PT_bNoGrip"
  spec_PT_rTrq/1 -> BC/2  "testSig_PT_rTrq"
  spec_CoETS_trqUnFltLtd/1 -> BC/3  "testSig_CoETS_trqUnFltLtd"
  spec_CoETS_trqInrLimSet/1 -> BC/4  "testSig_CoETS_trqInrLimSet"
  spec_ASDrf_trqInrSet/1 -> BC/5  "testSig_ASDrf_trqInrSet"
  spec_ASDdc_trq/1 -> BC/6  "testSig_ASDdc_trq"
  spec_CoEng_stShutOffPath/1 -> BC/7  "testSig_CoEng_stShutOffPath"
  spec_CoEng_st/1 -> BC/8  "testSig_CoEng_st"
  spec_StSys_trqStrt/1 -> BC/9  "testSig_StSys_trqStrt"
  spec_PthSet_stOvrRun/1 -> BC/10  "testSig_PthSet_stOvrRun"
  spec_EngTrqPtd_trqLim/1 -> BC/11  "testSig_EngTrqPtd_trqLim"
  spec_EngTrqPtd_stPthLim/1 -> BC/12  "testSig_EngTrqPtd_stPthLim"
  spec_PthSet_trqInrSetSum/1 -> BC/13  "testSig_PthSet_trqInrSetSum"
  spec_PthSet_stActvMonLim/1 -> BC/14  "testSig_PthSet_stActvMonLim"
  spec_PthSet_trqInrSet/1 -> BC/15  "testSig_PthSet_trqInrSet"

== system TST_PthSet_TrqCalc/simulationInput/testSignals_R004 ==
  BC : BusCreator  Inputs=15
  spec_ASDdc_trq : FromWorkspace  VariableName=testSig_ASDdc_trq  Interpolate=off  OutputAfterFinalValue=Holding final value
  spec_ASDrf_trqInrSet : FromWorkspace  VariableName=testSig_ASDrf_trqInrSet  Interpolate=off  OutputAfterFinalValue=Holding final value
  spec_CoETS_trqInrLimSet : FromWorkspace  VariableName=testSig_CoETS_trqInrLimSet  Interpolate=off  OutputAfterFinalValue=Holding final value
  spec_CoETS_trqUnFltLtd : FromWorkspace  VariableName=testSig_CoETS_trqUnFltLtd  Interpolate=off  OutputAfterFinalValue=Holding final value
  spec_CoEng_st : FromWorkspace  VariableName=testSig_CoEng_st  Interpolate=off  OutputAfterFinalValue=Holding final value
  spec_CoEng_stShutOffPath : FromWorkspace  VariableName=testSig_CoEng_stShutOffPath  Interpolate=off  OutputAfterFinalValue=Holding final value
  spec_EngTrqPtd_stPthLim : FromWorkspace  VariableName=testSig_EngTrqPtd_stPthLim  Interpolate=off  OutputAfterFinalValue=Holding final value
  spec_EngTrqPtd_trqLim : FromWorkspace  VariableName=testSig_EngTrqPtd_trqLim  Interpolate=off  OutputAfterFinalValue=Holding final value
  spec_PT_bNoGrip : FromWorkspace  VariableName=testSig_PT_bNoGrip  Interpolate=off  OutputAfterFinalValue=Holding final value
  spec_PT_rTrq : FromWorkspace  VariableName=testSig_PT_rTrq  Interpolate=off  OutputAfterFinalValue=Holding final value
  spec_PthSet_stActvMonLim : FromWorkspace  VariableName=testSig_PthSet_stActvMonLim  Interpolate=off  OutputAfterFinalValue=Holding final value
  spec_PthSet_stOvrRun : FromWorkspace  VariableName=testSig_PthSet_stOvrRun  Interpolate=off  OutputAfterFinalValue=Holding final value
  spec_PthSet_trqInrSet : FromWorkspace  VariableName=testSig_PthSet_trqInrSet  Interpolate=off  OutputAfterFinalValue=Holding final value
  spec_PthSet_trqInrSetSum : FromWorkspace  VariableName=testSig_PthSet_trqInrSetSum  Interpolate=off  OutputAfterFinalValue=Holding final value
  spec_StSys_trqStrt : FromWorkspace  VariableName=testSig_StSys_trqStrt  Interpolate=off  OutputAfterFinalValue=Holding final value
  testSignals : Outport
  wires:
  BC/1 -> testSignals/1
  spec_PT_bNoGrip/1 -> BC/1  "testSig_PT_bNoGrip"
  spec_PT_rTrq/1 -> BC/2  "testSig_PT_rTrq"
  spec_CoETS_trqUnFltLtd/1 -> BC/3  "testSig_CoETS_trqUnFltLtd"
  spec_CoETS_trqInrLimSet/1 -> BC/4  "testSig_CoETS_trqInrLimSet"
  spec_ASDrf_trqInrSet/1 -> BC/5  "testSig_ASDrf_trqInrSet"
  spec_ASDdc_trq/1 -> BC/6  "testSig_ASDdc_trq"
  spec_CoEng_stShutOffPath/1 -> BC/7  "testSig_CoEng_stShutOffPath"
  spec_CoEng_st/1 -> BC/8  "testSig_CoEng_st"
  spec_StSys_trqStrt/1 -> BC/9  "testSig_StSys_trqStrt"
  spec_PthSet_stOvrRun/1 -> BC/10  "testSig_PthSet_stOvrRun"
  spec_EngTrqPtd_trqLim/1 -> BC/11  "testSig_EngTrqPtd_trqLim"
  spec_EngTrqPtd_stPthLim/1 -> BC/12  "testSig_EngTrqPtd_stPthLim"
  spec_PthSet_trqInrSetSum/1 -> BC/13  "testSig_PthSet_trqInrSetSum"
  spec_PthSet_stActvMonLim/1 -> BC/14  "testSig_PthSet_stActvMonLim"
  spec_PthSet_trqInrSet/1 -> BC/15  "testSig_PthSet_trqInrSet"

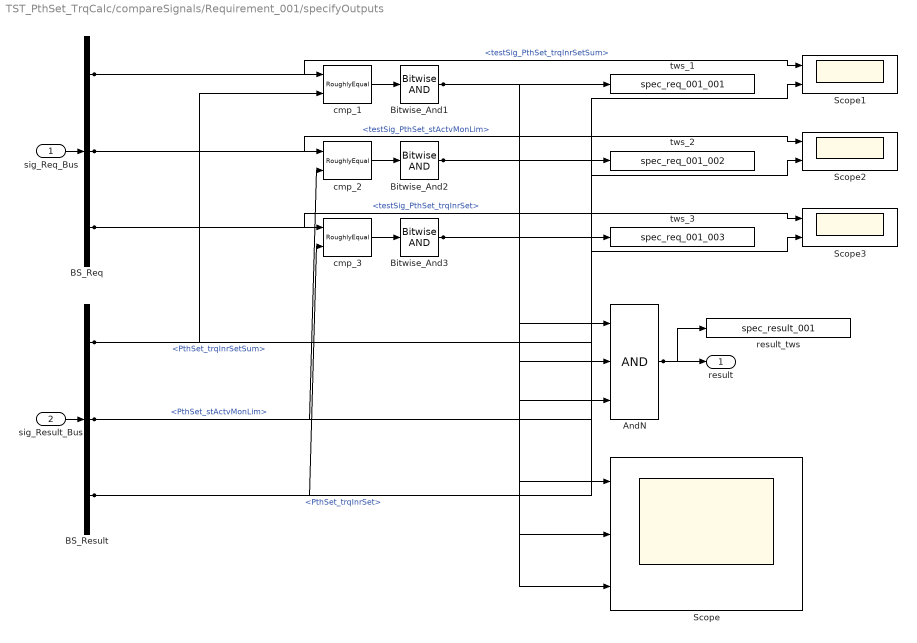
== system TST_PthSet_TrqCalc/compareSignals/Requirement_001/specifyOutputs ==
  sig_Req_Bus : Inport
  sig_Result_Bus : Inport  Port=2
  AndN : Logic  Inputs=3
  BS_Req : BusSelector  OutputSignals=testSig_PthSet_trqInrSetSum,testSig_PthSet_stActvMonLim,testSig_PthSet_trqInrSet
  BS_Result : BusSelector  OutputSignals=PthSet_trqInrSetSum,PthSet_stActvMonLim,PthSet_trqInrSet
  Bitwise_And1 : simulink/Logic and Bit Operations/Bitwise Operator  logicop=AND  UseBitMask=off  BitMask=bin2dec('11011001')  BitMaskRealWorld=Stored Integer
  Bitwise_And2 : simulink/Logic and Bit Operations/Bitwise Operator  logicop=AND  UseBitMask=off  BitMask=bin2dec('11011001')  BitMaskRealWorld=Stored Integer
  Bitwise_And3 : simulink/Logic and Bit Operations/Bitwise Operator  logicop=AND  UseBitMask=off  BitMask=bin2dec('11011001')  BitMaskRealWorld=Stored Integer
  Scope : Scope  NumInputPorts=3
  Scope1 : Scope  NumInputPorts=2
  Scope2 : Scope  NumInputPorts=2
  Scope3 : Scope  NumInputPorts=2
  cmp_1 : UnitTest_Lib/RoughlyEqual  slope=0.1
  cmp_2 : UnitTest_Lib/RoughlyEqual  slope=0.1
  cmp_3 : UnitTest_Lib/RoughlyEqual  slope=0.1
  result_tws : ToWorkspace  VariableName=spec_result_001
  tws_1 : ToWorkspace  VariableName=spec_req_001_001
  tws_2 : ToWorkspace  VariableName=spec_req_001_002
  tws_3 : ToWorkspace  VariableName=spec_req_001_003
  result : Outport
  wires:
  sig_Req_Bus/1 -> BS_Req/1
  sig_Result_Bus/1 -> BS_Result/1
  AndN/1 -> result/1, result_tws/1
  BS_Req/1 -> cmp_1/1, Scope1/1  "<testSig_PthSet_trqInrSetSum>"
  BS_Result/1 -> cmp_1/2, Scope1/2  "<PthSet_trqInrSetSum>"
  cmp_1/1 -> Bitwise_And1/1
  Bitwise_And1/1 -> tws_1/1, AndN/1, Scope/1
  BS_Req/2 -> cmp_2/1, Scope2/1  "<testSig_PthSet_stActvMonLim>"
  BS_Result/2 -> cmp_2/2, Scope2/2  "<PthSet_stActvMonLim>"
  cmp_2/1 -> Bitwise_And2/1
  Bitwise_And2/1 -> tws_2/1, AndN/2, Scope/2
  BS_Req/3 -> cmp_3/1, Scope3/1  "<testSig_PthSet_trqInrSet>"
  BS_Result/3 -> cmp_3/2, Scope3/2  "<PthSet_trqInrSet>"
  cmp_3/1 -> Bitwise_And3/1
  Bitwise_And3/1 -> tws_3/1, AndN/3, Scope/3

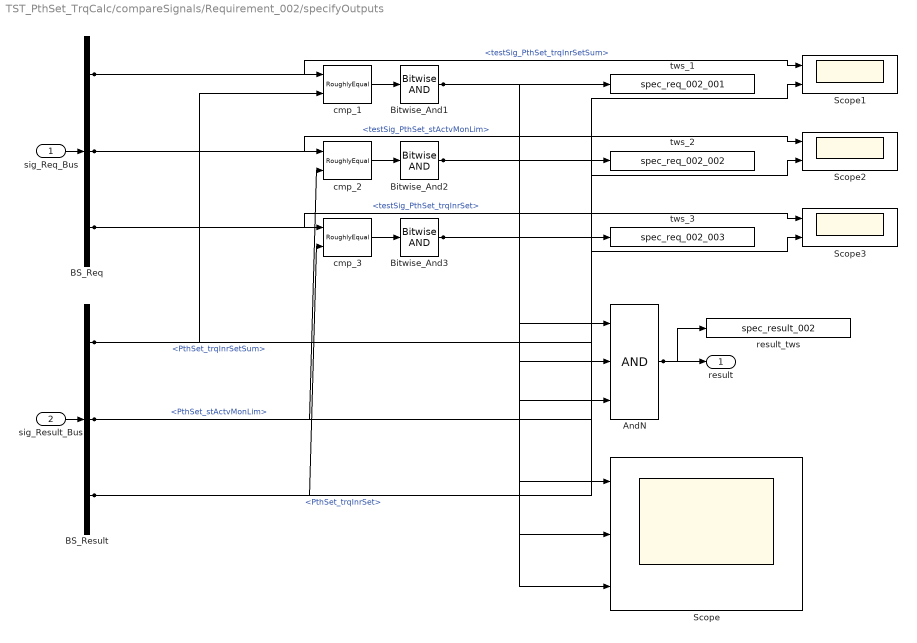
== system TST_PthSet_TrqCalc/compareSignals/Requirement_002/specifyOutputs ==
  sig_Req_Bus : Inport
  sig_Result_Bus : Inport  Port=2
  AndN : Logic  Inputs=3
  BS_Req : BusSelector  OutputSignals=testSig_PthSet_trqInrSetSum,testSig_PthSet_stActvMonLim,testSig_PthSet_trqInrSet
  BS_Result : BusSelector  OutputSignals=PthSet_trqInrSetSum,PthSet_stActvMonLim,PthSet_trqInrSet
  Bitwise_And1 : simulink/Logic and Bit Operations/Bitwise Operator  logicop=AND  UseBitMask=off  BitMask=bin2dec('11011001')  BitMaskRealWorld=Stored Integer
  Bitwise_And2 : simulink/Logic and Bit Operations/Bitwise Operator  logicop=AND  UseBitMask=off  BitMask=bin2dec('11011001')  BitMaskRealWorld=Stored Integer
  Bitwise_And3 : simulink/Logic and Bit Operations/Bitwise Operator  logicop=AND  UseBitMask=off  BitMask=bin2dec('11011001')  BitMaskRealWorld=Stored Integer
  Scope : Scope  NumInputPorts=3
  Scope1 : Scope  NumInputPorts=2
  Scope2 : Scope  NumInputPorts=2
  Scope3 : Scope  NumInputPorts=2
  cmp_1 : UnitTest_Lib/RoughlyEqual  slope=0.1
  cmp_2 : UnitTest_Lib/RoughlyEqual  slope=0.1
  cmp_3 : UnitTest_Lib/RoughlyEqual  slope=0.1
  result_tws : ToWorkspace  VariableName=spec_result_002
  tws_1 : ToWorkspace  VariableName=spec_req_002_001
  tws_2 : ToWorkspace  VariableName=spec_req_002_002
  tws_3 : ToWorkspace  VariableName=spec_req_002_003
  result : Outport
  wires:
  sig_Req_Bus/1 -> BS_Req/1
  sig_Result_Bus/1 -> BS_Result/1
  AndN/1 -> result/1, result_tws/1
  BS_Req/1 -> cmp_1/1, Scope1/1  "<testSig_PthSet_trqInrSetSum>"
  BS_Result/1 -> cmp_1/2, Scope1/2  "<PthSet_trqInrSetSum>"
  cmp_1/1 -> Bitwise_And1/1
  Bitwise_And1/1 -> tws_1/1, AndN/1, Scope/1
  BS_Req/2 -> cmp_2/1, Scope2/1  "<testSig_PthSet_stActvMonLim>"
  BS_Result/2 -> cmp_2/2, Scope2/2  "<PthSet_stActvMonLim>"
  cmp_2/1 -> Bitwise_And2/1
  Bitwise_And2/1 -> tws_2/1, AndN/2, Scope/2
  BS_Req/3 -> cmp_3/1, Scope3/1  "<testSig_PthSet_trqInrSet>"
  BS_Result/3 -> cmp_3/2, Scope3/2  "<PthSet_trqInrSet>"
  cmp_3/1 -> Bitwise_And3/1
  Bitwise_And3/1 -> tws_3/1, AndN/3, Scope/3

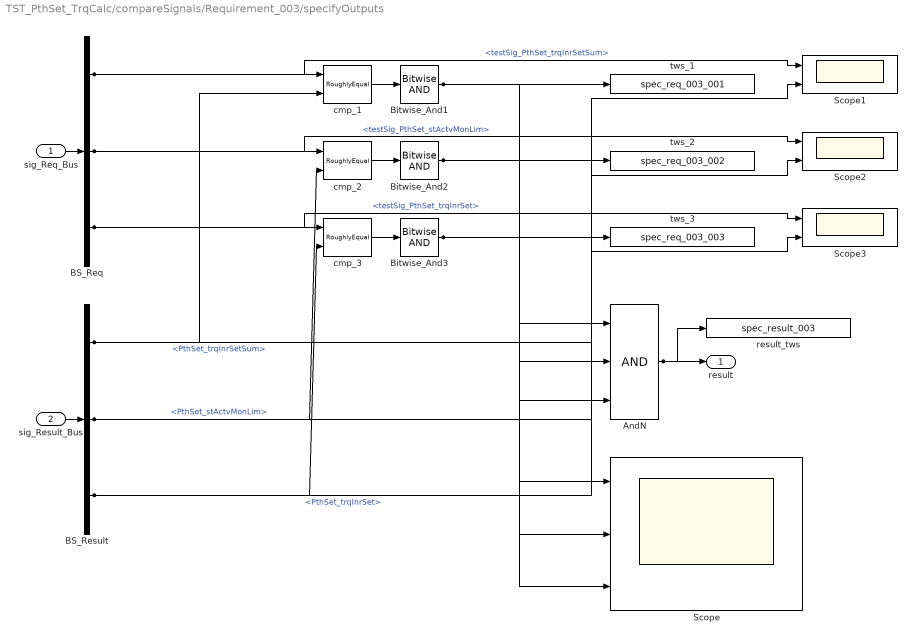
== system TST_PthSet_TrqCalc/compareSignals/Requirement_003/specifyOutputs ==
  sig_Req_Bus : Inport
  sig_Result_Bus : Inport  Port=2
  AndN : Logic  Inputs=3
  BS_Req : BusSelector  OutputSignals=testSig_PthSet_trqInrSetSum,testSig_PthSet_stActvMonLim,testSig_PthSet_trqInrSet
  BS_Result : BusSelector  OutputSignals=PthSet_trqInrSetSum,PthSet_stActvMonLim,PthSet_trqInrSet
  Bitwise_And1 : simulink/Logic and Bit Operations/Bitwise Operator  logicop=AND  UseBitMask=off  BitMask=bin2dec('11011001')  BitMaskRealWorld=Stored Integer
  Bitwise_And2 : simulink/Logic and Bit Operations/Bitwise Operator  logicop=AND  UseBitMask=off  BitMask=bin2dec('11011001')  BitMaskRealWorld=Stored Integer
  Bitwise_And3 : simulink/Logic and Bit Operations/Bitwise Operator  logicop=AND  UseBitMask=off  BitMask=bin2dec('11011001')  BitMaskRealWorld=Stored Integer
  Scope : Scope  NumInputPorts=3
  Scope1 : Scope  NumInputPorts=2
  Scope2 : Scope  NumInputPorts=2
  Scope3 : Scope  NumInputPorts=2
  cmp_1 : UnitTest_Lib/RoughlyEqual  slope=0.1
  cmp_2 : UnitTest_Lib/RoughlyEqual  slope=0.1
  cmp_3 : UnitTest_Lib/RoughlyEqual  slope=0.1
  result_tws : ToWorkspace  VariableName=spec_result_003
  tws_1 : ToWorkspace  VariableName=spec_req_003_001
  tws_2 : ToWorkspace  VariableName=spec_req_003_002
  tws_3 : ToWorkspace  VariableName=spec_req_003_003
  result : Outport
  wires:
  sig_Req_Bus/1 -> BS_Req/1
  sig_Result_Bus/1 -> BS_Result/1
  AndN/1 -> result/1, result_tws/1
  BS_Req/1 -> cmp_1/1, Scope1/1  "<testSig_PthSet_trqInrSetSum>"
  BS_Result/1 -> cmp_1/2, Scope1/2  "<PthSet_trqInrSetSum>"
  cmp_1/1 -> Bitwise_And1/1
  Bitwise_And1/1 -> tws_1/1, AndN/1, Scope/1
  BS_Req/2 -> cmp_2/1, Scope2/1  "<testSig_PthSet_stActvMonLim>"
  BS_Result/2 -> cmp_2/2, Scope2/2  "<PthSet_stActvMonLim>"
  cmp_2/1 -> Bitwise_And2/1
  Bitwise_And2/1 -> tws_2/1, AndN/2, Scope/2
  BS_Req/3 -> cmp_3/1, Scope3/1  "<testSig_PthSet_trqInrSet>"
  BS_Result/3 -> cmp_3/2, Scope3/2  "<PthSet_trqInrSet>"
  cmp_3/1 -> Bitwise_And3/1
  Bitwise_And3/1 -> tws_3/1, AndN/3, Scope/3

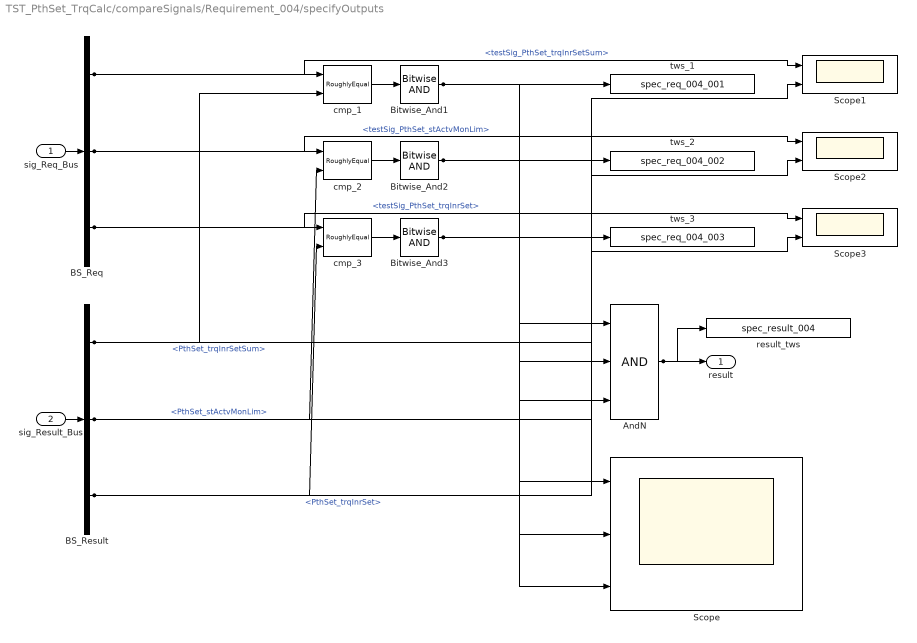
== system TST_PthSet_TrqCalc/compareSignals/Requirement_004/specifyOutputs ==
  sig_Req_Bus : Inport
  sig_Result_Bus : Inport  Port=2
  AndN : Logic  Inputs=3
  BS_Req : BusSelector  OutputSignals=testSig_PthSet_trqInrSetSum,testSig_PthSet_stActvMonLim,testSig_PthSet_trqInrSet
  BS_Result : BusSelector  OutputSignals=PthSet_trqInrSetSum,PthSet_stActvMonLim,PthSet_trqInrSet
  Bitwise_And1 : simulink/Logic and Bit Operations/Bitwise Operator  logicop=AND  UseBitMask=off  BitMask=bin2dec('11011001')  BitMaskRealWorld=Stored Integer
  Bitwise_And2 : simulink/Logic and Bit Operations/Bitwise Operator  logicop=AND  UseBitMask=off  BitMask=bin2dec('11011001')  BitMaskRealWorld=Stored Integer
  Bitwise_And3 : simulink/Logic and Bit Operations/Bitwise Operator  logicop=AND  UseBitMask=off  BitMask=bin2dec('11011001')  BitMaskRealWorld=Stored Integer
  Scope : Scope  NumInputPorts=3
  Scope1 : Scope  NumInputPorts=2
  Scope2 : Scope  NumInputPorts=2
  Scope3 : Scope  NumInputPorts=2
  cmp_1 : UnitTest_Lib/RoughlyEqual  slope=0.1
  cmp_2 : UnitTest_Lib/RoughlyEqual  slope=0.1
  cmp_3 : UnitTest_Lib/RoughlyEqual  slope=0.1
  result_tws : ToWorkspace  VariableName=spec_result_004
  tws_1 : ToWorkspace  VariableName=spec_req_004_001
  tws_2 : ToWorkspace  VariableName=spec_req_004_002
  tws_3 : ToWorkspace  VariableName=spec_req_004_003
  result : Outport
  wires:
  sig_Req_Bus/1 -> BS_Req/1
  sig_Result_Bus/1 -> BS_Result/1
  AndN/1 -> result/1, result_tws/1
  BS_Req/1 -> cmp_1/1, Scope1/1  "<testSig_PthSet_trqInrSetSum>"
  BS_Result/1 -> cmp_1/2, Scope1/2  "<PthSet_trqInrSetSum>"
  cmp_1/1 -> Bitwise_And1/1
  Bitwise_And1/1 -> tws_1/1, AndN/1, Scope/1
  BS_Req/2 -> cmp_2/1, Scope2/1  "<testSig_PthSet_stActvMonLim>"
  BS_Result/2 -> cmp_2/2, Scope2/2  "<PthSet_stActvMonLim>"
  cmp_2/1 -> Bitwise_And2/1
  Bitwise_And2/1 -> tws_2/1, AndN/2, Scope/2
  BS_Req/3 -> cmp_3/1, Scope3/1  "<testSig_PthSet_trqInrSet>"
  BS_Result/3 -> cmp_3/2, Scope3/2  "<PthSet_trqInrSet>"
  cmp_3/1 -> Bitwise_And3/1
  Bitwise_And3/1 -> tws_3/1, AndN/3, Scope/3
